simulink model "test"  (R2017b)
settings: Solver=VariableStepAuto  StartTime=0.0  StopTime=3  RelTol=1e-3
libraries: simulink x2
settings Model: Creator=Administrator  LastModifiedBy=Administrator

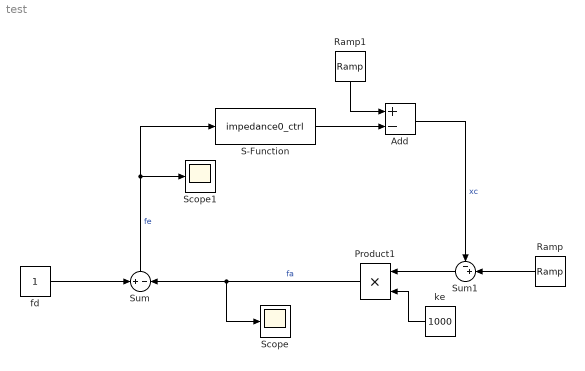
== system test ==
  Add : Sum  Inputs=+-
  Product1 : Product
  Ramp : simulink/Sources/Ramp  slope=1  start=0  X0=0
  Ramp1 : simulink/Sources/Ramp  slope=1  start=0  X0=-1
  S-Function : S-Function  FunctionName=impedance0_ctrl  SFunctionDeploymentMode=off  EnableBusSupport=off
  Scope : Scope
  Scope1 : Scope
  Sum : Sum  Inputs=+|-
  Sum1 : Sum  Inputs=-+|
  fd : Constant
  ke : Constant  Value=1000
  wires:
  S-Function/1 -> Add/2
  Ramp1/1 -> Add/1
  Add/1 -> Sum1/1  "xc"
  Ramp/1 -> Sum1/2
  Sum1/1 -> Product1/1
  ke/1 -> Product1/2
  Product1/1 -> Scope/1, Sum/2  "fa"
  fd/1 -> Sum/1
  Sum/1 -> Scope1/1, S-Function/1  "fe"
